simulink model "derivador_discreto"  (R2023b)
settings: Solver=VariableStepAuto  StartTime=0.0  StopTime=0.01  RelTol=1e-3
values from neighbouring files (symbols this model uses):
  Ts = interp_ts(Ts_ts,t)    [calcular_metricas_operacion.m]
settings Model: Creator=Pc  LastModifiedBy=Pc

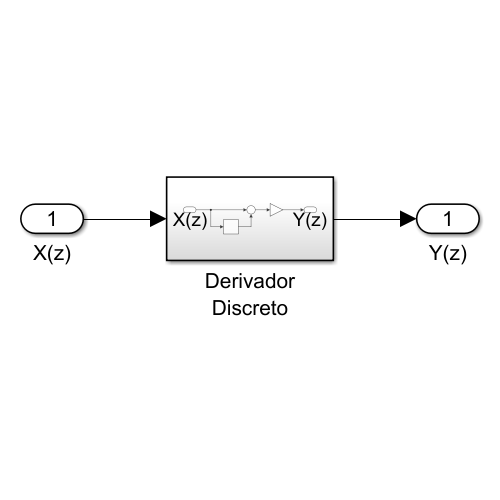
[thumbnail: Simulink's stored preview of the top-level diagram]
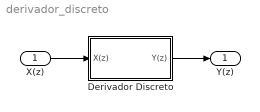
== system derivador_discreto ==
  X(z) : Inport
  Derivador Discreto : Subsystem
  Y(z) : Outport
  wires:
  X(z)/1 -> Derivador Discreto/1(X(z))
  Derivador Discreto/1(Y(z)) -> Y(z)/1

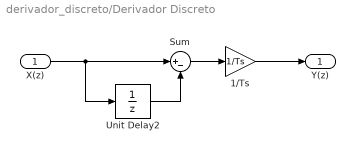
== system derivador_discreto/Derivador Discreto ==
  X(z) : Inport
  1/Ts : Gain  Gain=1/Ts
  Sum : Sum  Inputs=|+-
  Unit Delay2 : UnitDelay  SampleTime=Ts  HasFrameUpgradeWarning=on
  Y(z) : Outport
  wires:
  Unit Delay2/1 -> Sum/2
  X(z)/1 -> Sum/1, Unit Delay2/1
  1/Ts/1 -> Y(z)/1
  Sum/1 -> 1/Ts/1
